simulink model "APNG"  (Simulink 7.1)
settings: Solver=ode45  StartTime=0.0  StopTime=40  MaxStep=0.001  RelTol=1e-3
values from neighbouring files (symbols this model uses):
  AT = 3    [linearizedPNG_ini.m]    (also in missdisatnce_adjoint.m; missdistance_homing_loop.m; missdistance_linearized.m; truePNG_ini.m = 0)
  BETA_INI = (90 * pi/180)    (= 1.57079632679)    [truePNG_ini.m]
  GUIDE_SEL = 1    [OGL_ini.m]    (also in truePNG_ini.m)
  LOS_INI = atan2(YT_INI-YM_INI , XT_INI-XM_INI )    [truePNG_ini.m]
  MAX_ACC = 7    [linearizedPNG_ini.m]    (also in truePNG_ini.m = 0.5)
  RTOL = 0.01    [truePNG_ini.m]
  Tautopilot = 0    [linearizedPNG_ini.m]    (also in missdisatnce_adjoint.m = 2; missdistance_homing_loop.m = 2; missdistance_linearized.m = 2; truePNG_ini.m = 0.2)
  VT = 40    [linearizedPNG_ini.m]    (also in truePNG_ini.m = 0.25)
  VXM_INI = VM * cos(GAMMA_INI)    [truePNG_ini.m]
  VYM_INI = VM * sin(GAMMA_INI)    [truePNG_ini.m]
  XM_INI = -1    [truePNG_ini.m]
  XT_INI = 1    [truePNG_ini.m]
  YM_INI = -1    [truePNG_ini.m]
  YT_INI = -1    [truePNG_ini.m]
libraries: simulink x1
settings Model: Creator=Lorenzo  LastModifiedBy=LESSONS
settings DebuggingCC: SaveWithParameterizedLinksMsg=none
settings GRTTargetCC: TargetFcnLib=ansi_tfl_tmw.mat

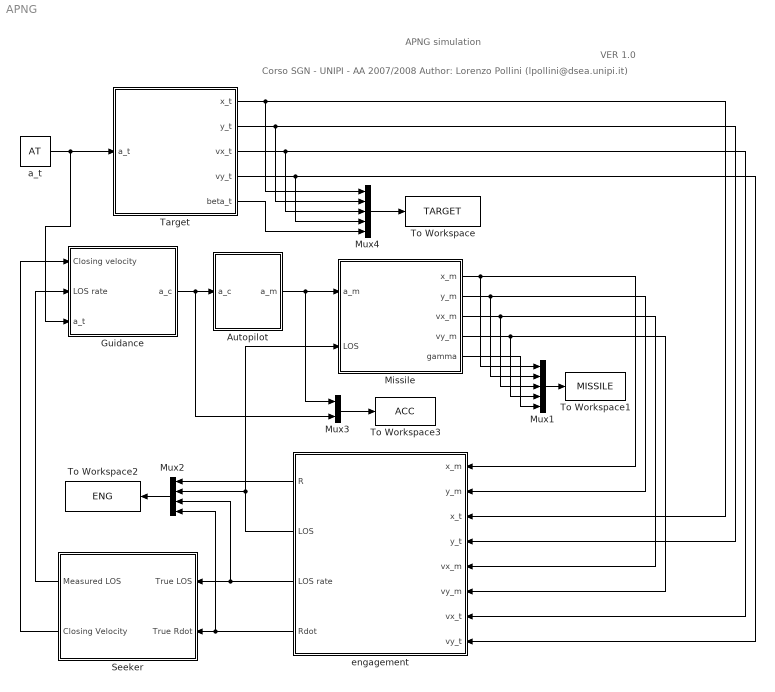
== system APNG ==
  note: APNG simulation
  note: Corso SGN - UNIPI - AA 2007/2008
      | Author: Lorenzo Pollini (lpollini@dsea.unipi.it)
  note: VER 1.0
  Autopilot : Subsystem
  Guidance : Subsystem
  Missile : Subsystem
  Mux1 : Mux  Inputs=5
  Mux2 : Mux  Orientation=left
  Mux3 : Mux  Inputs=2
  Mux4 : Mux  Inputs=5
  Seeker : Subsystem  Orientation=left
  Target : Subsystem
  To Workspace : ToWorkspace  VariableName=TARGET  SampleTime=-1  SaveFormat=Structure With Time
  To Workspace1 : ToWorkspace  VariableName=MISSILE  SampleTime=-1  SaveFormat=Structure With Time
  To Workspace2 : ToWorkspace  VariableName=ENG  SampleTime=-1  SaveFormat=Structure With Time
  To Workspace3 : ToWorkspace  VariableName=ACC  SampleTime=-1  SaveFormat=Structure With Time
  a_t : Constant  Value=AT  OutDataType=sfix(16)  OutScaling=2^0
  engagement : Subsystem  Orientation=left
  wires:
  Target/1(x_t) -> engagement/3(x_t), Mux4/1
  Target/2(y_t) -> engagement/4(y_t), Mux4/2
  Target/3(vx_t) -> engagement/7(vx_t), Mux4/3
  Target/4(vy_t) -> engagement/8(vy_t), Mux4/4
  Missile/1(x_m) -> engagement/1(x_m), Mux1/1
  Missile/2(y_m) -> engagement/2(y_m), Mux1/2
  Missile/3(vx_m) -> engagement/5(vx_m), Mux1/3
  Missile/4(vy_m) -> Mux1/4, engagement/6(vy_m)
  engagement/2(LOS) -> Missile/2(LOS), Mux2/2
  engagement/3(LOS rate) -> Mux2/3, Seeker/1(True LOS)
  engagement/4(Rdot) -> Mux2/4, Seeker/2(True Rdot)
  Seeker/2(Closing Velocity) -> Guidance/1(Closing velocity)
  Guidance/1(a_c) -> Autopilot/1(a_c), Mux3/2
  Mux4/1 -> To Workspace/1
  Mux1/1 -> To Workspace1/1
  Mux2/1 -> To Workspace2/1
  engagement/1(R) -> Mux2/1
  Seeker/1(Measured LOS) -> Guidance/2(LOS rate)
  Autopilot/1(a_m) -> Missile/1(a_m), Mux3/1
  Missile/5(gamma) -> Mux1/5
  Mux3/1 -> To Workspace3/1
  Target/5(beta_t) -> Mux4/5
  a_t/1 -> Target/1(a_t), Guidance/3(a_t)

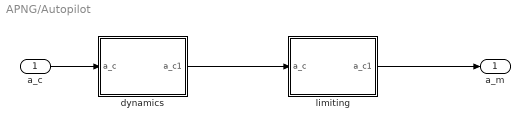
== system APNG/Autopilot ==
  a_c : Inport  OutDataType=sfix(16)  OutScaling=2^0
  dynamics : Subsystem
  limiting : Subsystem
  a_m : Outport  OutDataType=sfix(16)  OutScaling=2^0
  wires:
  a_c/1 -> dynamics/1(a_c)
  dynamics/1(a_c1) -> limiting/1(a_c)
  limiting/1(a_c1) -> a_m/1

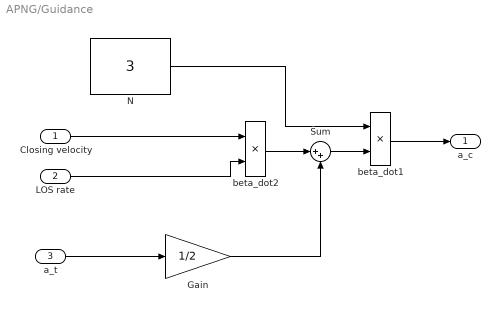
== system APNG/Guidance ==
  Closing velocity : Inport  OutDataType=sfix(16)  OutScaling=2^0
  LOS rate : Inport  Port=2  OutDataType=sfix(16)  OutScaling=2^0
  a_t : Inport  Port=3  OutDataType=sfix(16)  OutScaling=2^0
  Gain : Gain  Gain=1/2  ParameterDataType=sfix(16)  ParameterScaling=2^0  OutDataType=sfix(16)  OutScaling=2^0
  N : Constant  Value=3  OutDataType=sfix(16)  OutScaling=2^0
  Sum : Sum  Inputs=|++  OutDataType=sfix(16)  OutScaling=2^0
  beta_dot1 : Product  Inputs=**  OutDataType=sfix(16)  OutScaling=2^-10
  beta_dot2 : Product  Inputs=**  OutDataType=sfix(16)  OutScaling=2^-10
  a_c : Outport  OutDataType=sfix(16)  OutScaling=2^0
  wires:
  Closing velocity/1 -> beta_dot2/1
  LOS rate/1 -> beta_dot2/2
  N/1 -> beta_dot1/1
  a_t/1 -> Gain/1
  beta_dot1/1 -> a_c/1
  beta_dot2/1 -> Sum/1
  Sum/1 -> beta_dot1/2
  Gain/1 -> Sum/2

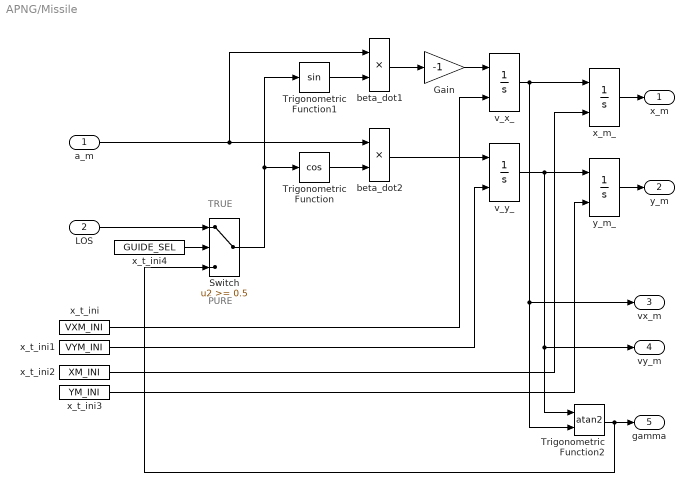
== system APNG/Missile ==
  note: TRUE
  note: PURE
  a_m : Inport  OutDataType=sfix(16)  OutScaling=2^0
  LOS : Inport  Port=2  OutDataType=sfix(16)  OutScaling=2^0
  Gain : Gain  Gain=-1  ParameterDataType=sfix(16)  ParameterScaling=2^0  OutDataType=sfix(16)  OutScaling=2^0
  Switch : Switch  Threshold=0.5
  Trigonometric Function : Trigonometry  Operator=cos
  Trigonometric Function1 : Trigonometry
  Trigonometric Function2 : Trigonometry  Operator=atan2
  beta_dot1 : Product  Inputs=**  OutDataType=sfix(16)  OutScaling=2^-10
  beta_dot2 : Product  Inputs=**  OutDataType=sfix(16)  OutScaling=2^-10
  v_x_ : Integrator  InitialConditionSource=external
  v_y_ : Integrator  InitialConditionSource=external
  x_m_ : Integrator  InitialConditionSource=external
  x_t_ini : Constant  Value=VXM_INI  OutDataType=sfix(16)  OutScaling=2^0
  x_t_ini1 : Constant  Value=VYM_INI  OutDataType=sfix(16)  OutScaling=2^0
  x_t_ini2 : Constant  Value=XM_INI  OutDataType=sfix(16)  OutScaling=2^0
  x_t_ini3 : Constant  Value=YM_INI  OutDataType=sfix(16)  OutScaling=2^0
  x_t_ini4 : Constant  Value=GUIDE_SEL  OutDataType=sfix(16)  OutScaling=2^0
  y_m_ : Integrator  InitialConditionSource=external
  x_m : Outport  OutDataType=sfix(16)  OutScaling=2^0
  y_m : Outport  Port=2  OutDataType=sfix(16)  OutScaling=2^0
  vx_m : Outport  Port=3  OutDataType=sfix(16)  OutScaling=2^0
  vy_m : Outport  Port=4  OutDataType=sfix(16)  OutScaling=2^0
  gamma : Outport  Port=5  OutDataType=sfix(16)  OutScaling=2^0
  wires:
  Trigonometric Function/1 -> beta_dot2/2
  beta_dot1/1 -> Gain/1
  Trigonometric Function1/1 -> beta_dot1/2
  y_m_/1 -> y_m/1
  x_m_/1 -> x_m/1
  v_x_/1 -> x_m_/1, vx_m/1, Trigonometric Function2/2
  v_y_/1 -> y_m_/1, vy_m/1, Trigonometric Function2/1
  Gain/1 -> v_x_/1
  a_m/1 -> beta_dot1/1, beta_dot2/1
  beta_dot2/1 -> v_y_/1
  x_t_ini/1 -> v_x_/2
  x_t_ini1/1 -> v_y_/2
  x_t_ini2/1 -> x_m_/2
  x_t_ini3/1 -> y_m_/2
  Trigonometric Function2/1 -> gamma/1, Switch/3
  LOS/1 -> Switch/1
  Switch/1 -> Trigonometric Function1/1, Trigonometric Function/1
  x_t_ini4/1 -> Switch/2

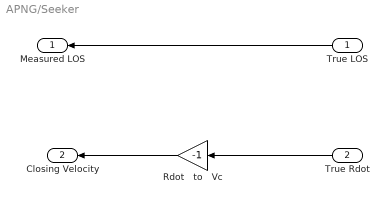
== system APNG/Seeker ==
  True LOS : Inport  Orientation=left  OutDataType=sfix(16)  OutScaling=2^0
  True Rdot : Inport  Orientation=left  Port=2  OutDataType=sfix(16)  OutScaling=2^0
  Rdot   to   Vc : Gain  Orientation=left  Gain=-1  ParameterDataType=sfix(16)  ParameterScaling=2^0  OutDataType=sfix(16)  OutScaling=2^0
  Measured LOS : Outport  Orientation=left  OutDataType=sfix(16)  OutScaling=2^0
  Closing Velocity : Outport  Orientation=left  Port=2  OutDataType=sfix(16)  OutScaling=2^0
  wires:
  True LOS/1 -> Measured LOS/1
  Rdot   to   Vc/1 -> Closing Velocity/1
  True Rdot/1 -> Rdot   to   Vc/1

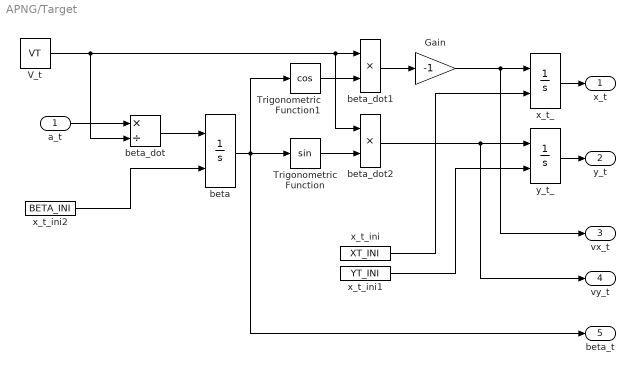
== system APNG/Target ==
  a_t : Inport  OutDataType=sfix(16)  OutScaling=2^0
  Gain : Gain  Gain=-1  ParameterDataType=sfix(16)  ParameterScaling=2^0  OutDataType=sfix(16)  OutScaling=2^0
  Trigonometric Function : Trigonometry
  Trigonometric Function1 : Trigonometry  Operator=cos
  V_t : Constant  Value=VT  OutDataType=sfix(16)  OutScaling=2^0
  beta : Integrator  InitialConditionSource=external
  beta_dot : Product  Inputs=*/  OutDataType=sfix(16)  OutScaling=2^-10
  beta_dot1 : Product  Inputs=**  OutDataType=sfix(16)  OutScaling=2^-10
  beta_dot2 : Product  Inputs=**  OutDataType=sfix(16)  OutScaling=2^-10
  x_t_ : Integrator  InitialConditionSource=external
  x_t_ini : Constant  Value=XT_INI  OutDataType=sfix(16)  OutScaling=2^0
  x_t_ini1 : Constant  Value=YT_INI  OutDataType=sfix(16)  OutScaling=2^0
  x_t_ini2 : Constant  Value=BETA_INI  OutDataType=sfix(16)  OutScaling=2^0
  y_t_ : Integrator  InitialConditionSource=external
  x_t : Outport  OutDataType=sfix(16)  OutScaling=2^0
  y_t : Outport  Port=2  OutDataType=sfix(16)  OutScaling=2^0
  vx_t : Outport  Port=3  OutDataType=sfix(16)  OutScaling=2^0
  vy_t : Outport  Port=4  OutDataType=sfix(16)  OutScaling=2^0
  beta_t : Outport  Port=5  OutDataType=sfix(16)  OutScaling=2^0
  wires:
  V_t/1 -> beta_dot1/1, beta_dot2/1, beta_dot/2
  beta_dot/1 -> beta/1
  beta/1 -> Trigonometric Function/1, Trigonometric Function1/1, beta_t/1
  x_t_ini2/1 -> beta/2
  x_t_/1 -> x_t/1
  y_t_/1 -> y_t/1
  Trigonometric Function1/1 -> beta_dot1/2
  beta_dot1/1 -> Gain/1
  Trigonometric Function/1 -> beta_dot2/2
  beta_dot2/1 -> y_t_/1, vy_t/1
  Gain/1 -> x_t_/1, vx_t/1
  x_t_ini1/1 -> y_t_/2
  x_t_ini/1 -> x_t_/2
  a_t/1 -> beta_dot/1

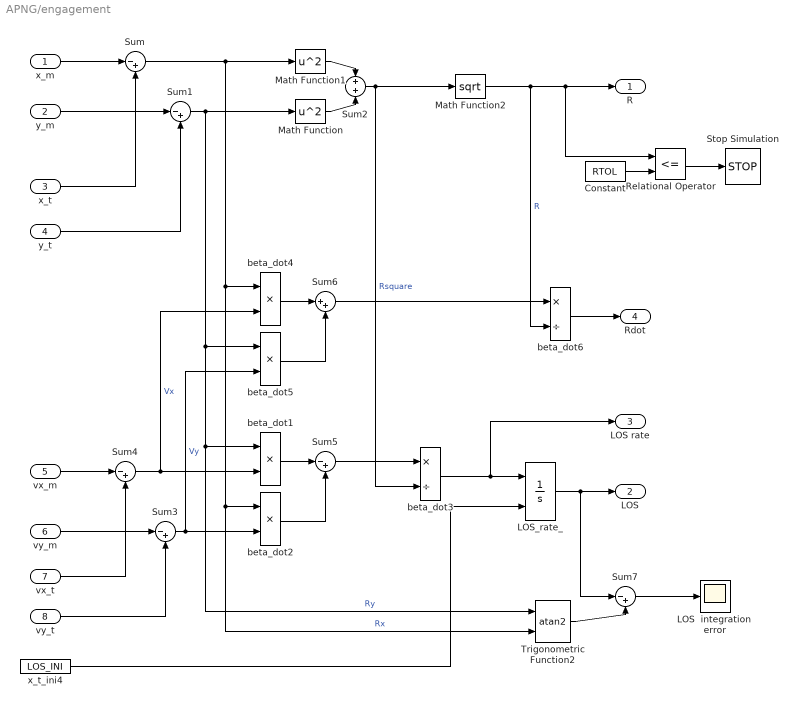
== system APNG/engagement ==
  x_m : Inport  OutDataType=sfix(16)  OutScaling=2^0
  y_m : Inport  Port=2  OutDataType=sfix(16)  OutScaling=2^0
  x_t : Inport  Port=3  OutDataType=sfix(16)  OutScaling=2^0
  y_t : Inport  Port=4  OutDataType=sfix(16)  OutScaling=2^0
  vx_m : Inport  Port=5  OutDataType=sfix(16)  OutScaling=2^0
  vy_m : Inport  Port=6  OutDataType=sfix(16)  OutScaling=2^0
  vx_t : Inport  Port=7  OutDataType=sfix(16)  OutScaling=2^0
  vy_t : Inport  Port=8  OutDataType=sfix(16)  OutScaling=2^0
  Constant : Constant  Value=RTOL  OutDataType=sfix(16)  OutScaling=2^0
  LOS  integration  error : Scope
  LOS_rate_ : Integrator  InitialConditionSource=external
  Math Function : Math  Operator=square  OutDataType=sfix(16)  OutScaling=2^0  SaturateOnIntegerOverflow=on
  Math Function1 : Math  Operator=square  OutDataType=sfix(16)  OutScaling=2^0  SaturateOnIntegerOverflow=on
  Math Function2 : Math  Operator=sqrt  OutDataType=sfix(16)  OutScaling=2^0  SaturateOnIntegerOverflow=on
  Relational Operator : RelationalOperator  Operator=<=  LogicOutDataTypeMode=boolean  OutDataTypeStr=boolean
  Stop Simulation : Stop
  Sum{,1,3..5,7} (6 alike) : Sum  Inputs=|-+  OutDataType=sfix(16)  OutScaling=2^0
  Sum2 : Sum  Inputs=+|+  OutDataType=sfix(16)  OutScaling=2^0
  Sum6 : Sum  Inputs=|++  OutDataType=sfix(16)  OutScaling=2^0
  Trigonometric Function2 : Trigonometry  Operator=atan2
  beta_dot{1..2,4..5} (4 alike) : Product  Inputs=**  OutDataType=sfix(16)  OutScaling=2^-10
  beta_dot3 : Product  Inputs=*/  OutDataType=sfix(16)  OutScaling=2^-10
  beta_dot6 : Product  Inputs=*/  OutDataType=sfix(16)  OutScaling=2^-10
  x_t_ini4 : Constant  Value=LOS_INI  OutDataType=sfix(16)  OutScaling=2^0
  R : Outport  OutDataType=sfix(16)  OutScaling=2^0
  LOS : Outport  Port=2  OutDataType=sfix(16)  OutScaling=2^0
  LOS rate : Outport  Port=3  OutDataType=sfix(16)  OutScaling=2^0
  Rdot : Outport  Port=4  OutDataType=sfix(16)  OutScaling=2^0
  wires:
  x_t_ini4/1 -> LOS_rate_/2
  x_m/1 -> Sum/1
  x_t/1 -> Sum/2
  y_m/1 -> Sum1/1
  y_t/1 -> Sum1/2
  Sum/1 -> Math Function1/1, beta_dot4/1, beta_dot2/1, Trigonometric Function2/2  "Rx"
  Sum1/1 -> Math Function/1, beta_dot5/1, beta_dot1/1, Trigonometric Function2/1  "Ry"
  Math Function1/1 -> Sum2/1
  Math Function/1 -> Sum2/2
  Sum2/1 -> Math Function2/1, beta_dot3/2  "Rsquare"
  Math Function2/1 -> beta_dot6/2, R/1, Relational Operator/1  "R"
  vx_m/1 -> Sum4/1
  vx_t/1 -> Sum4/2
  vy_m/1 -> Sum3/1
  vy_t/1 -> Sum3/2
  Sum4/1 -> beta_dot1/2, beta_dot4/2  "Vx"
  Sum3/1 -> beta_dot2/2, beta_dot5/2  "Vy"
  beta_dot1/1 -> Sum5/1
  beta_dot2/1 -> Sum5/2
  Sum5/1 -> beta_dot3/1
  beta_dot3/1 -> LOS_rate_/1, LOS rate/1
  LOS_rate_/1 -> LOS/1, Sum7/1
  beta_dot4/1 -> Sum6/1
  beta_dot5/1 -> Sum6/2
  Sum6/1 -> beta_dot6/1
  beta_dot6/1 -> Rdot/1
  Constant/1 -> Relational Operator/2
  Relational Operator/1 -> Stop Simulation/1
  Trigonometric Function2/1 -> Sum7/2
  Sum7/1 -> LOS  integration  error/1

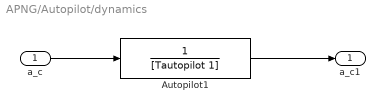
== system APNG/Autopilot/dynamics ==
  a_c : Inport  OutDataType=sfix(16)  OutScaling=2^0
  Autopilot1 : TransferFcn  Denominator=[Tautopilot 1]
  a_c1 : Outport  OutDataType=sfix(16)  OutScaling=2^0
  wires:
  a_c/1 -> Autopilot1/1
  Autopilot1/1 -> a_c1/1

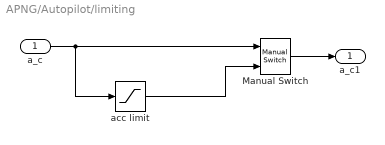
== system APNG/Autopilot/limiting ==
  a_c : Inport  OutDataType=sfix(16)  OutScaling=2^0
  Manual Switch : simulink/Signal Routing/Manual Switch  SystemSampleTime=-1  sw=1  action=0  varsize=off
  acc limit : Saturate  UpperLimit=MAX_ACC  LowerLimit=-MAX_ACC
  a_c1 : Outport  OutDataType=sfix(16)  OutScaling=2^0
  wires:
  Manual Switch/1 -> a_c1/1
  a_c/1 -> Manual Switch/1, acc limit/1
  acc limit/1 -> Manual Switch/2
